simulink model "sl_quadcopter_ss"  (Simulink 8.3)
settings: Solver=ode45  StartTime=0.0  StopTime=20  MaxStep=0.1  RelTol=1e-3
InitFcn:
  | % load parameters of the default quadrotor
  | disp('Quadrotor parameters loaded by InitFcn')
  | mdl_quadcopter
undefined symbols (not defined in the file or in its folder): quad
libraries: roblocks x3
settings Model: Creator=corkep  LastModifiedBy=matteo
settings OptimizationCC: ExpressionDepthLimit=2147483647
settings DebuggingCC: FcnCallInpInsideContextMsg=EnableAllAsWarning

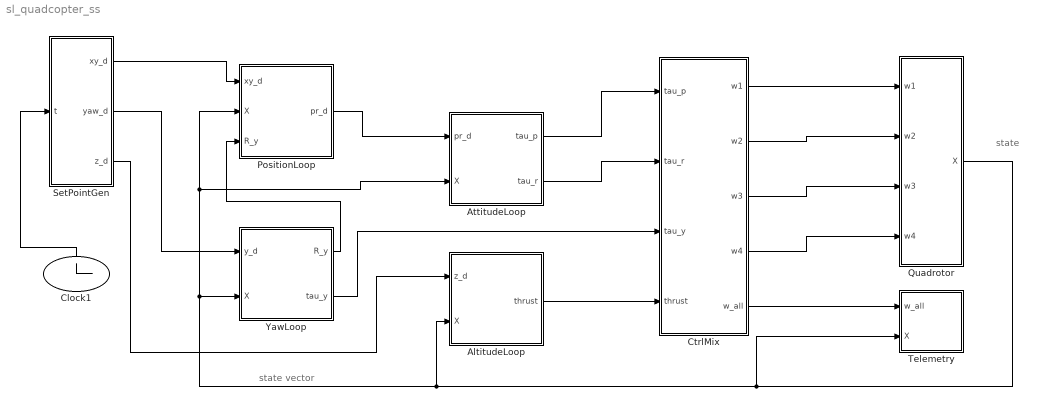
== system sl_quadcopter_ss ==
  note: state
  note: state vector
  AltitudeLoop : Subsystem
  AttitudeLoop : Subsystem
  Clock1 : Clock
  CtrlMix : Subsystem
  PositionLoop : Subsystem
  Quadrotor : Subsystem
  SetPointGen : Subsystem
  Telemetry : Subsystem
  YawLoop : Subsystem
  wires:
  SetPointGen/1(xy_d) -> PositionLoop/1(xy_d)
  PositionLoop/1(pr_d) -> AttitudeLoop/1(pr_d)
  YawLoop/2(tau_y) -> CtrlMix/3(tau_y)
  SetPointGen/3(z_d) -> AltitudeLoop/1(z_d)
  AttitudeLoop/2(tau_r) -> CtrlMix/2(tau_r)
  CtrlMix/5(w_all) -> Telemetry/1(w_all)
  SetPointGen/2(yaw_d) -> YawLoop/1(y_d)
  YawLoop/1(R_y) -> PositionLoop/3(R_y)
  AttitudeLoop/1(tau_p) -> CtrlMix/1(tau_p)
  AltitudeLoop/1(thrust) -> CtrlMix/4(thrust)
  Clock1/1 -> SetPointGen/1(t)
  Quadrotor/1(X) -> YawLoop/2(X), AttitudeLoop/2(X), PositionLoop/2(X), AltitudeLoop/2(X), Telemetry/2(X)
  CtrlMix/1(w1) -> Quadrotor/1(w1)
  CtrlMix/2(w2) -> Quadrotor/2(w2)
  CtrlMix/3(w3) -> Quadrotor/3(w3)
  CtrlMix/4(w4) -> Quadrotor/4(w4)

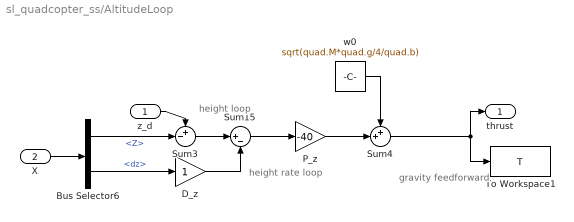
== system sl_quadcopter_ss/AltitudeLoop ==
  note: gravity feedforward
  note: height rate
      | loop
  note: height
      | loop
  z_d : Inport
  X : Inport  Port=2
  Bus Selector6 : BusSelector  OutputSignals=Z,dz
  D_z : Gain
  P_z : Gain  Gain=-40
  Sum15 : Sum  Inputs=|+-
  Sum3 : Sum  Inputs=+-|
  Sum4 : Sum  Inputs=++|
  To Workspace1 : ToWorkspace  VariableName=T  SampleTime=-1
  w0 : Constant  Value=sqrt(quad.M*quad.g/4/quad.b)  SampleTime=0
  thrust : Outport
  wires:
  w0/1 -> Sum4/1
  Sum15/1 -> P_z/1
  P_z/1 -> Sum4/2
  Bus Selector6/1 -> Sum3/2  "<Z>"
  Sum3/1 -> Sum15/1
  Bus Selector6/2 -> D_z/1  "<dz>"
  D_z/1 -> Sum15/2
  Sum4/1 -> To Workspace1/1, thrust/1
  X/1 -> Bus Selector6/1
  z_d/1 -> Sum3/1

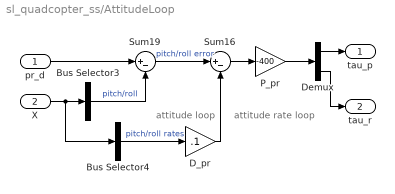
== system sl_quadcopter_ss/AttitudeLoop ==
  note: attitude rate
      | loop
  note: attitude
      | loop
  pr_d : Inport
  X : Inport  Port=2
  Bus Selector3 : BusSelector  OutputSignals=pitch,roll  OutputAsBus=on
  Bus Selector4 : BusSelector  OutputSignals=dpitch,droll  OutputAsBus=on
  D_pr : Gain  Gain=.1
  Demux : Demux  Outputs=2
  P_pr : Gain  Gain=-400
  Sum16 : Sum  Inputs=|+-
  Sum19 : Sum  Inputs=|+-
  tau_p : Outport
  tau_r : Outport  Port=2
  wires:
  Bus Selector3/1 -> Sum19/2  "pitch/roll"
  Bus Selector4/1 -> D_pr/1  "pitch/roll rates"
  Sum19/1 -> Sum16/1  "pitch/roll error"
  Sum16/1 -> P_pr/1
  P_pr/1 -> Demux/1
  D_pr/1 -> Sum16/2
  X/1 -> Bus Selector3/1, Bus Selector4/1
  Demux/1 -> tau_p/1
  pr_d/1 -> Sum19/1
  Demux/2 -> tau_r/1

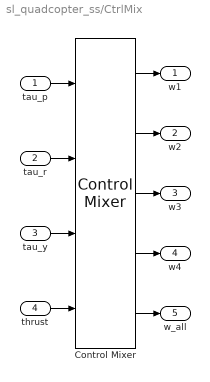
== system sl_quadcopter_ss/CtrlMix ==
  tau_p : Inport
  tau_r : Inport  Port=2
  tau_y : Inport  Port=3
  thrust : Inport  Port=4
  Control Mixer : roblocks/Dynamics/Control Mixer
  w1 : Outport
  w2 : Outport  Port=2
  w3 : Outport  Port=3
  w4 : Outport  Port=4
  w_all : Outport  Port=5
  wires:
  Control Mixer/1 -> w1/1
  tau_p/1 -> Control Mixer/1
  Control Mixer/2 -> w2/1
  tau_r/1 -> Control Mixer/2
  Control Mixer/3 -> w3/1
  tau_y/1 -> Control Mixer/3
  Control Mixer/4 -> w4/1
  thrust/1 -> Control Mixer/4
  Control Mixer/5 -> w_all/1

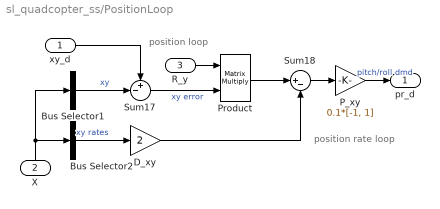
== system sl_quadcopter_ss/PositionLoop ==
  note: position rate
      | loop
  note: position
      | loop
  xy_d : Inport
  X : Inport  Port=2
  R_y : Inport  Port=3
  Bus Selector1 : BusSelector  OutputSignals=X,Y  OutputAsBus=on
  Bus Selector2 : BusSelector  OutputSignals=dx,dy  OutputAsBus=on
  D_xy : Gain  Gain=2
  P_xy : Gain  Gain=0.1*[-1, 1]
  Product : Product  Multiplication=Matrix(*)  RndMeth=Zero
  Sum17 : Sum  Inputs=+-|
  Sum18 : Sum  Inputs=|+-
  pr_d : Outport
  wires:
  Bus Selector1/1 -> Sum17/2  "xy"
  Bus Selector2/1 -> D_xy/1  "xy rates"
  D_xy/1 -> Sum18/2
  Sum18/1 -> P_xy/1
  Product/1 -> Sum18/1
  Sum17/1 -> Product/2  "xy error"
  X/1 -> Bus Selector1/1, Bus Selector2/1
  R_y/1 -> Product/1
  xy_d/1 -> Sum17/1
  P_xy/1 -> pr_d/1  "pitch/roll dmd"

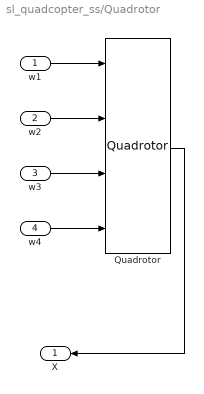
== system sl_quadcopter_ss/Quadrotor ==
  w1 : Inport
  w2 : Inport  Port=2
  w3 : Inport  Port=3
  w4 : Inport  Port=4
  Quadrotor : roblocks/Dynamics/Quadrotor  quad=quad
  X : Outport
  wires:
  w1/1 -> Quadrotor/1
  w4/1 -> Quadrotor/4
  Quadrotor/1 -> X/1
  w3/1 -> Quadrotor/3
  w2/1 -> Quadrotor/2

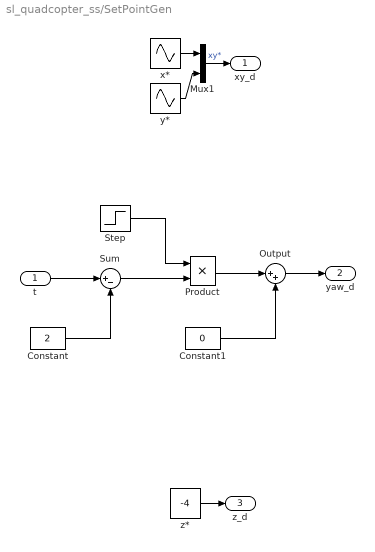
== system sl_quadcopter_ss/SetPointGen ==
  t : Inport
  Constant : Constant  DisableCoverage=on  Value=2  OutDataTypeStr=Inherit: Inherit via back propagation
  Constant1 : Constant  DisableCoverage=on  Value=0  OutDataTypeStr=Inherit: Inherit via back propagation
  Mux1 : Mux  Inputs=2
  Output : Sum  Inputs=|++  SaturateOnIntegerOverflow=on  InputSameDT=on  OutDataTypeStr=Inherit: Same as first input
  Product : Product  DisableCoverage=on  SaturateOnIntegerOverflow=on  InputSameDT=on  OutDataTypeStr=Inherit: Same as first input
  Step : Step  DisableCoverage=on  Time=2  After=0.2  SampleTime=0
  Sum : Sum  DisableCoverage=on  Inputs=|+-  SaturateOnIntegerOverflow=on  InputSameDT=on  OutDataTypeStr=Inherit: Same as first input
  x* : Sin  Frequency=2*pi*.125  Phase=-pi/2  SampleTime=0
  y* : Sin  Frequency=2*pi*.125  SampleTime=0
  z* : Constant  Value=-4  SampleTime=0
  xy_d : Outport
  yaw_d : Outport  Port=2
  z_d : Outport  Port=3
  wires:
  x*/1 -> Mux1/1
  y*/1 -> Mux1/2
  Mux1/1 -> xy_d/1  "xy*"
  z*/1 -> z_d/1
  t/1 -> Sum/1
  Constant/1 -> Sum/2
  Sum/1 -> Product/2
  Output/1 -> yaw_d/1
  Constant1/1 -> Output/2
  Product/1 -> Output/1
  Step/1 -> Product/1

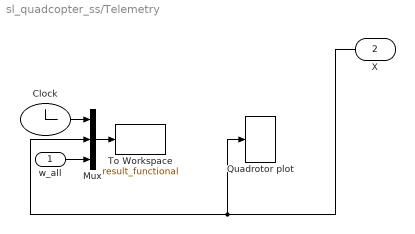
== system sl_quadcopter_ss/Telemetry ==
  w_all : Inport
  X : Inport  Port=2
  Clock : Clock
  Mux : Mux  Inputs=3
  Quadrotor plot : roblocks/Robot Graphics/Quadrotor plot  x=0
  To Workspace : ToWorkspace  VariableName=result_functional  SampleTime=0.05
  wires:
  Mux/1 -> To Workspace/1
  Clock/1 -> Mux/1
  X/1 -> Quadrotor plot/1, Mux/2
  w_all/1 -> Mux/3

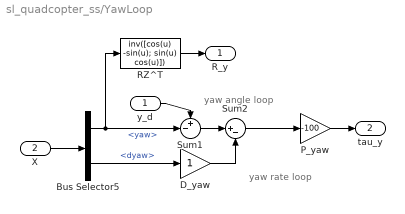
== system sl_quadcopter_ss/YawLoop ==
  note: yaw rate
      | loop
  note: yaw angle
      | loop
  y_d : Inport
  X : Inport  Port=2
  Bus Selector5 : BusSelector  OutputSignals=yaw,dyaw
  D_yaw : Gain
  P_yaw : Gain  Gain=-100
  RZ^T : MATLABFcn  MATLABFcn=inv([cos(u) -sin(u); sin(u) cos(u)])  OutputDimensions=[2 2]  Output1D=off
  Sum1 : Sum  Inputs=+-|
  Sum2 : Sum  Inputs=|+-
  R_y : Outport
  tau_y : Outport  Port=2
  wires:
  Bus Selector5/1 -> RZ^T/1, Sum1/2  "<yaw>"
  Sum2/1 -> P_yaw/1
  Bus Selector5/2 -> D_yaw/1  "<dyaw>"
  D_yaw/1 -> Sum2/2
  Sum1/1 -> Sum2/1
  X/1 -> Bus Selector5/1
  RZ^T/1 -> R_y/1
  y_d/1 -> Sum1/1
  P_yaw/1 -> tau_y/1
